simulink model "refroidissement_copy"  (R2019b)
settings: Solver=FixedStepAuto  StartTime=0.0  StopTime=inf  FixedStep=0.01  RelTol=1e-3
libraries: arduinolib x13, dspstat3 x6, simulink x2, LCDlib x1, Laboratoire x1
settings Model: SILPILModeSetting=veronly  ExtModeTrigDuration=2  Creator=Guy  LastModifiedBy=Etudiant
settings OptimizationCC: PassReuseOutputArgsAs=Individual arguments  ZeroExternalMemoryAtStartup=off  ZeroInternalMemoryAtStartup=off  MaxStackSize=64  OptimizeBlockOrder=speed  EfficientTunableParamExpr=on
settings DebuggingCC: ParameterTunabilityLossMsg=error
settings HardwareCC: ProdBitPerInt=16  ProdBitPerPointer=16  ProdBitPerSizeT=16  ProdBitPerPtrDiffT=16  ProdLargestAtomicFloat=None  ProdWordSize=8  ProdHWDeviceType=Atmel->AVR
settings SFSimCC: MATLABDynamicMemAlloc=off
settings RTWCC: SystemTargetFile=ert.tlc  HardwareBoard=Arduino Mega 2560  TLCOptions=-aInlineSetEventsForThisBaseRateFcn=TLC_FALSE -aSuppressMultiTaskScheduler=TLC_FALSE -aRateBasedStepFcn=1  TemplateMakefile=ert_default_tmf  CustomSource=enc_eml_src.c  Toolchain=Arduino AVR  BuildConfiguration=Faster Runs  IncludeHyperlinkInReport=on
settings CodeAppCC: ForceParamTrailComments=on  GenerateComments=off  IgnoreCustomStorageClasses=off  OperatorAnnotations=on  SimulinkDataObjDesc=on  SFDataObjDesc=on  InsertBlockDesc=on
settings ERTTargetCC: SupportContinuousTime=on  SupportVariableSizeSignals=on  ExtModeStaticAllocSize=2048

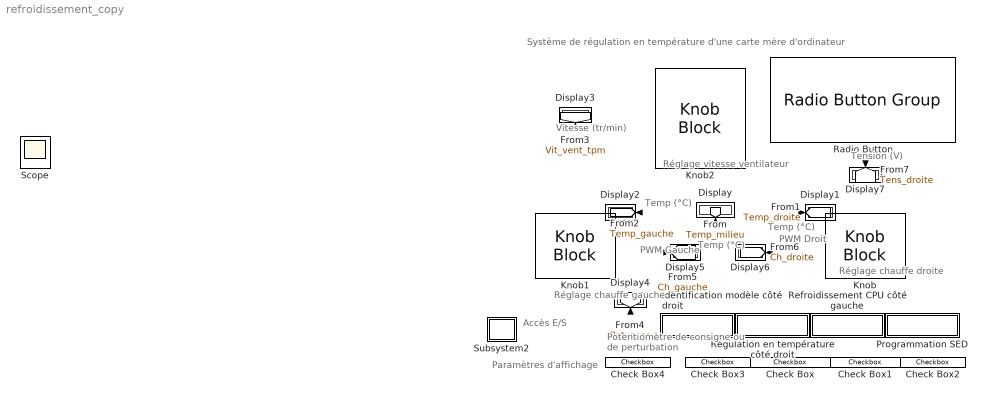
== system refroidissement_copy ==
  note: Paramètres d'affichage
  note: PWM
      | Gauche
  note: Système de régulation en température d'une carte mère d'ordinateur
  note: PWM
      | Droit
  note: Tension (V)
  note: Temp (°C)
  note: Temp (°C)
  note: Temp (°C)
  note: Vitesse (tr/min)
  note: Réglage vitesse ventilateur
  note: Réglage chauffe
      | droite
  note: Réglage chauffe
      | gauche
  note: Accès
      | E/S
  note: Potentiomètre
      | de consigne
      | ou de perturbation
  Check Box : Checkbox  LabelPosition=Hide  ShowInitialText=on  Label=Température gauche
  Check Box1 : Checkbox  LabelPosition=Hide  ShowInitialText=on  Label=Température milieu
  Check Box2 : Checkbox  LabelPosition=Hide  ShowInitialText=on  Label=Température droite
  Check Box3 : Checkbox  LabelPosition=Hide  ShowInitialText=on  Label=Tension résistance droite
  Check Box4 : Checkbox  LabelPosition=Hide  ShowInitialText=on  Label=Vitesse ventilateur (PWM)
  Display{,1..7} (8 alike) : Display
      Display3 settings: Decimation=20
  Identification modèle côté droit : Subsystem
  Knob : KnobBlock  LabelPosition=Hide  ScaleMax=255
  Knob1 : KnobBlock  LabelPosition=Hide  ScaleMax=255
  Knob2 : KnobBlock  LabelPosition=Hide  ScaleMax=255
  Programmation SED : Subsystem
  Radio Button : RadioButtonGroup  LabelPosition=Hide  SelectedLabel=Refroidissement CPU côté gauche  ButtonGroupName=Modes de marche
      settings: Values={{'Contrôle manuel', 'Régulation en température côté droit', 'Refroidissement CPU côté gauche', 'Programmation SED', 'Identification modèle côté droit', 'Arrêt'}, [0 1 2 3 4 5]}
  Refroidissement CPU côté gauche : Subsystem
  Régulation en température côté droit : Subsystem
  Subsystem2 : Subsystem
  Scope : Scope
  wires:
  [Temp_milieu] -> Display/1
  [Temp_droite] -> Display1/1
  [Temp_gauche] -> Display2/1
  [Vit_vent_tpm] -> Display3/1
  [Pot_cons] -> Display4/1
  [Ch_gauche] -> Display5/1
  [Ch_droite] -> Display6/1
  [Tens_droite] -> Display7/1

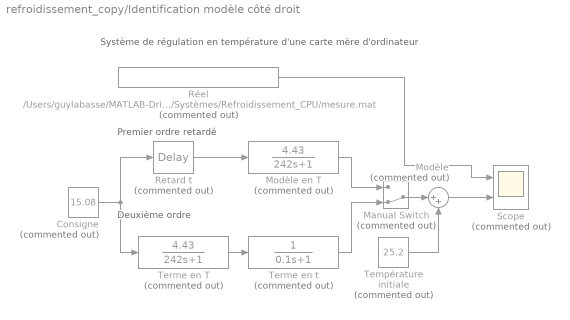
== system refroidissement_copy/Identification modèle côté droit ==
  note: Système de régulation en température d'une carte mère d'ordinateur
  note: Deuxième ordre
  note: Premier ordre retardé
  Consigne : Constant  Commented=on  Value=15.08
  Manual Switch : ManualSwitch  Commented=on  CurrentSetting=0
  Modèle : Sum  Commented=on  Inputs=|++
  Modèle en T : TransferFcn  Commented=on  Numerator=[4.43]  Denominator=[242 1]
  Retard t : TransportDelay  Commented=on  DelayTime=0.1
  Réel : FromFile  Commented=on  FileName=/Users/guylabasse/MATLAB-Drive/Systèmes/Refroidissement_CPU/mesure.mat  SampleTime=0.01
  Scope : Scope  Commented=on  NumInputPorts=2
  Température initiale : Constant  Commented=on  Value=25.2
  Terme en T : TransferFcn  Commented=on  Numerator=[4.43]  Denominator=[242 1]
  Terme en t : TransferFcn  Commented=on  Denominator=[0.1 1]
  wires:
  Consigne/1 -> Retard t/1, Terme en T/1
  Terme en T/1 -> Terme en t/1
  Température initiale/1 -> Modèle/2
  Terme en t/1 -> Manual Switch/2
  Modèle en T/1 -> Manual Switch/1
  Réel/1 -> Scope/1
  Manual Switch/1 -> Modèle/1
  Modèle/1 -> Scope/2
  Retard t/1 -> Modèle en T/1

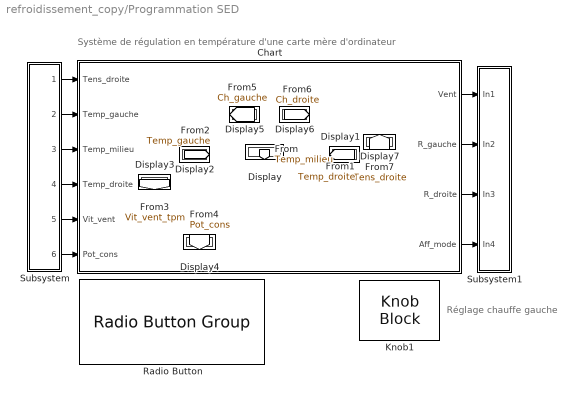
== system refroidissement_copy/Programmation SED ==
  note: Système de régulation en température d'une carte mère d'ordinateur
  note: Réglage chauffe
      | gauche
  Chart : Stateflow chart  BlockKeywords=__PRM__SERIALIZED__DATA__:Stateflow Chart,Stateflow Diagram  TreatAsAtomicUnit=on
  Display{,1..7} (8 alike) : Display
      Display3 settings: Decimation=20
  Knob1 : KnobBlock  LabelPosition=Hide  ScaleMax=250  TickInterval=50
  Radio Button : RadioButtonGroup  LabelPosition=Hide  SelectedLabel=Régulation en température côté gauche  ButtonGroupName=Modes de marche
      settings: Values={{'Contrôle manuel', 'Régulation en température côté droit', 'Régulation en température côté gauche', 'Programmation SED', 'Identification modèle côté droit', 'Arrêt'}, [0 1 2 3 4 5]}
  Subsystem : Subsystem
  Subsystem1 : Subsystem
  wires:
  [Temp_milieu] -> Display/1
  [Vit_vent_tpm] -> Display3/1
  [Tens_droite] -> Display7/1
  [Pot_cons] -> Display4/1
  [Temp_droite] -> Display1/1
  [Temp_gauche] -> Display2/1
  [Ch_gauche] -> Display5/1
  [Ch_droite] -> Display6/1
  Subsystem/1(Out1) -> Chart/1(Tens_droite)
  Subsystem/2(Out2) -> Chart/2(Temp_gauche)
  Subsystem/3(Out3) -> Chart/3(Temp_milieu)
  Subsystem/4(Out4) -> Chart/4(Temp_droite)
  Subsystem/5(Out5) -> Chart/5(Vit_vent)
  Subsystem/6(Out6) -> Chart/6(Pot_cons)
  Chart/1(Vent) -> Subsystem1/1(In1)
  Chart/2(R_gauche) -> Subsystem1/2(In2)
  Chart/3(R_droite) -> Subsystem1/3(In3)
  Chart/4(Aff_mode) -> Subsystem1/4(In4)

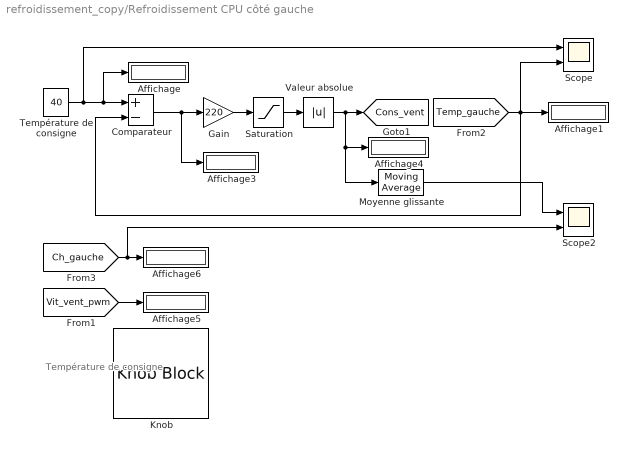
== system refroidissement_copy/Refroidissement CPU côté gauche ==
  note: Température
      | de consigne
  Affichage{,1,3..6} (6 alike) : Display
  Comparateur : Sum  Inputs=+-  OutDataTypeStr=double
  Gain : Gain  Gain=220
  Knob : KnobBlock  LabelPosition=Hide  TickInterval=10
  Moyenne glissante : dspstat3/Moving Average  Method=Sliding window  ForgettingFactorPort=off  SpecifyWindowLength=on  WindowLength=20  ForgettingFactor=0.9  SimulateUsing=Code generation
  Saturation : Saturate  UpperLimit=-81  LowerLimit=-10000
  Scope : Scope  NumInputPorts=2
  Scope2 : Scope  NumInputPorts=2
  Température de consigne : Constant  Value=40  SampleTime=-1
  Valeur absolue : Abs
  tag scope: Cons_vent=global
  wires:
  Température de consigne/1 -> Scope/1, Comparateur/1, Affichage/1
  Comparateur/1 -> Gain/1, Affichage3/1
  [Temp_gauche] -> Scope/2, Affichage1/1, Comparateur/2
  Gain/1 -> Saturation/1
  Valeur absolue/1 -> Affichage4/1, Moyenne glissante/1, [Cons_vent]
  [Vit_vent_pwm] -> Affichage5/1
  [Ch_gauche] -> Scope2/2, Affichage6/1
  Saturation/1 -> Valeur absolue/1
  Moyenne glissante/1 -> Scope2/1

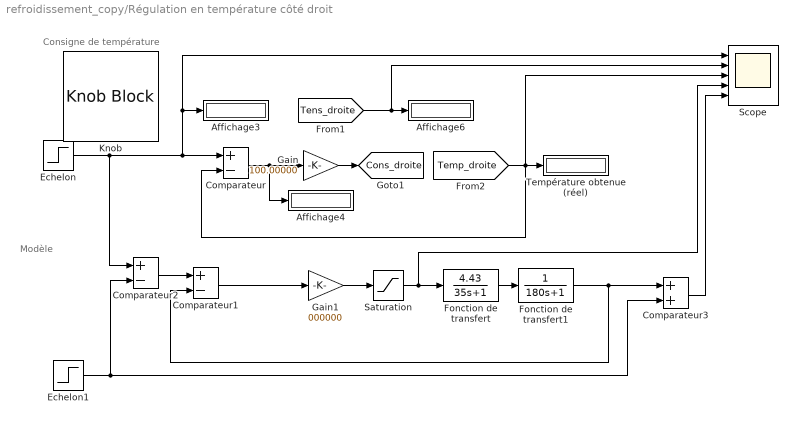
== system refroidissement_copy/Régulation en température côté droit ==
  note: Modèle
  note: Consigne de température
  Affichage3 : Display
  Affichage4 : Display
  Affichage6 : Display
  Comparateur : Sum  Inputs=+-  OutDataTypeStr=double
  Comparateur1 : Sum  Inputs=+-  OutDataTypeStr=double
  Comparateur2 : Sum  Inputs=+-  OutDataTypeStr=double
  Comparateur3 : Sum  OutDataTypeStr=double
  Echelon : Step  Time=0  After=0
  Echelon1 : Step  Time=10  After=0
  Fonction de transfert : TransferFcn  Numerator=[4.43]  Denominator=[35 1]
  Fonction de transfert1 : TransferFcn  Denominator=[180 1]
  Gain : Gain  Gain=100.00000
  Gain1 : Gain  Gain=000000
  Knob : KnobBlock  LabelPosition=Hide  TickInterval=20
  Saturation : Saturate  UpperLimit=15.08  LowerLimit=0
  Scope : Scope  NumInputPorts=5
  Température obtenue (réel) : Display
  tag scope: Cons_droite=global
  wires:
  [Tens_droite] -> Scope/2, Affichage6/1
  Echelon/1 -> Comparateur/1, Affichage3/1, Scope/1, Comparateur2/1
  [Temp_droite] -> Scope/3, Température obtenue (réel)/1, Comparateur/2
  Comparateur/1 -> Affichage4/1, Gain/1
  Gain/1 -> [Cons_droite]
  Comparateur1/1 -> Gain1/1
  Comparateur2/1 -> Comparateur1/1
  Echelon1/1 -> Comparateur3/2, Comparateur2/2
  Saturation/1 -> Scope/4, Fonction de transfert/1
  Fonction de transfert/1 -> Fonction de transfert1/1
  Fonction de transfert1/1 -> Comparateur1/2, Comparateur3/1
  Comparateur3/1 -> Scope/5
  Gain1/1 -> Saturation/1

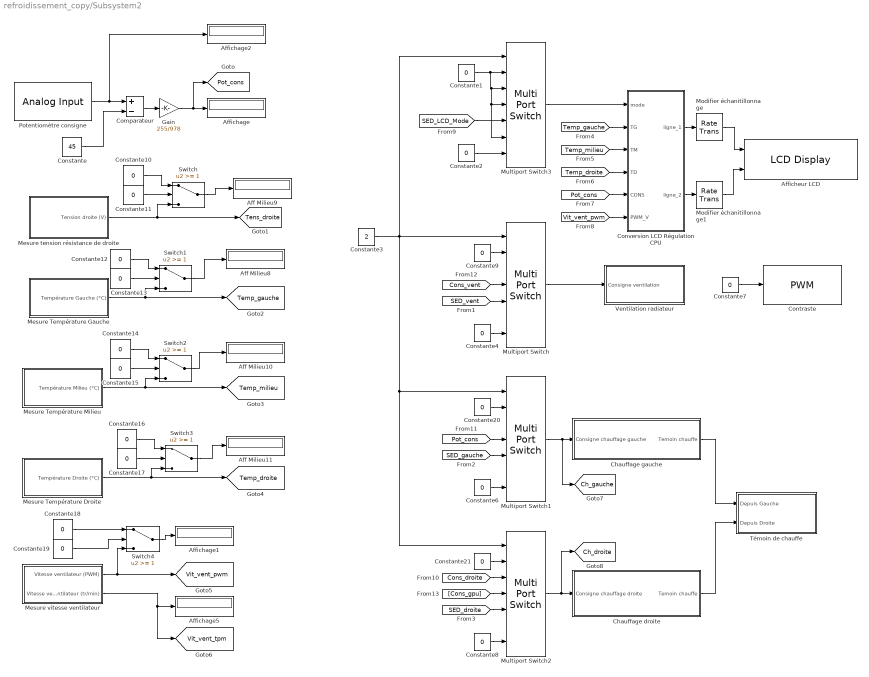
== system refroidissement_copy/Subsystem2 ==
  Aff Milieu{8..11} (4 alike) : Display
  Affichage{,1..2,5} (4 alike) : Display
  Afficheur LCD : LCDlib/LCD Display  pins=[30, 31, 32, 34, 36, 38]
      settings: SourceProductName=Arduino Extra Library
  Chauffage droite : Subsystem
  Chauffage gauche : Subsystem
  Comparateur : Sum  Inputs=+-  OutDataTypeStr=double
  Constante : Constant  Value=45  SampleTime=-1
  Constante{1..2,4,6,8..21} (18 alike) : Constant  Value=0  SampleTime=-1
  Constante3 : Constant  Value=2  SampleTime=-1
  Constante7 : Constant  Value=0  OutDataTypeStr=uint16  SampleTime=-1
  Contraste : arduinolib/PWM  pinNumber=44  EnableInputFrequency=off  InitialFrequency=2000  InitialDutyCycle=0  NotificationType=None  blockPlatform=arduino
  Conversion LCD Régulation CPU : MATLAB Function  TreatAsAtomicUnit=on
  Gain : Gain  Gain=255/978
  Mesure Température Droite : Subsystem
  Mesure Température Gauche : Subsystem
  Mesure Température Milieu : Subsystem
  Mesure tension résistance de droite : Subsystem
  Mesure vitesse ventilateur : Subsystem
  Modifier échanitillonnage : RateTransition  Integrity=off  OutPortSampleTime=1
  Modifier échanitillonnage1 : RateTransition  Integrity=off  OutPortSampleTime=1
  Multiport Switch{,1..3} (4 alike) : MultiPortSwitch  DataPortOrder=Zero-based contiguous  Inputs=6  DiagnosticForDefault=None  zeroidx=on  OutDataTypeStr=double
  Potentiomètre consigne : arduinolib/Analog Input  pinNumber=3  ReadResultsOnly=off  ConversionTriggerSource=Software  ExternalTriggerType=uint32(0)  OutputDataType=uint16  EnableConversionCompleteNotify=off  EnableOuputStatus=off  SampleTime=-1  blockPlatform=arduino
  Switch{,1..4} (5 alike) : Switch  Threshold=1
  Témoin de chauffe : Subsystem
  Ventilation radiateur : Subsystem
  tag scope: Ch_droite=global, Ch_gauche=global, Pot_cons=global, Temp_droite=global, Temp_gauche=global, Temp_milieu=global, Tens_droite=global, Vit_vent_pwm=global, Vit_vent_tpm=global
  wires:
  Modifier échanitillonnage1/1 -> Afficheur LCD/2
  Modifier échanitillonnage/1 -> Afficheur LCD/1
  Conversion LCD Régulation CPU/1(ligne_1) -> Modifier échanitillonnage/1
  Conversion LCD Régulation CPU/2(ligne_2) -> Modifier échanitillonnage1/1
  Mesure vitesse ventilateur/2(Vitesse ventilateur (tr/min)) -> [Vit_vent_tpm], Affichage5/1
  Mesure vitesse ventilateur/1(Vitesse ventilateur (PWM)) -> Switch4/3, [Vit_vent_pwm]
  Constante7/1 -> Contraste/1
  Multiport Switch/1 -> Ventilation radiateur/1(Consigne ventilation)
  Multiport Switch2/1 -> Chauffage droite/1(Consigne chauffage droite), [Ch_droite]
  Chauffage gauche/1(Temoin chauffe) -> Témoin de chauffe/1(Depuis Gauche)
  Multiport Switch1/1 -> [Ch_gauche], Chauffage gauche/1(Consigne chauffage gauche)
  Chauffage droite/1(Temoin chauffe) -> Témoin de chauffe/2(Depuis Droite)
  Gain/1 -> [Pot_cons], Affichage/1
  Switch/1 -> Aff Milieu9/1
  Mesure tension résistance de droite/1(Tension droite (V)) -> [Tens_droite], Switch/3
  Constante10/1 -> Switch/1
  Constante11/1 -> Switch/2
  Constante12/1 -> Switch1/1
  Constante13/1 -> Switch1/2
  Mesure Température Gauche/1(Température Gauche (°C)) -> [Temp_gauche], Switch1/3
  Switch1/1 -> Aff Milieu8/1
  Constante14/1 -> Switch2/1
  Constante15/1 -> Switch2/2
  Mesure Température Milieu/1(Température Milieu (°C)) -> [Temp_milieu], Switch2/3
  Switch2/1 -> Aff Milieu10/1
  Constante16/1 -> Switch3/1
  Constante17/1 -> Switch3/2
  Mesure Température Droite/1(Température Droite (°C)) -> [Temp_droite], Switch3/3
  Switch3/1 -> Aff Milieu11/1
  Constante18/1 -> Switch4/1
  Constante19/1 -> Switch4/2
  Switch4/1 -> Affichage1/1
  Constante4/1 -> Multiport Switch/7
  Constante6/1 -> Multiport Switch1/7
  Constante8/1 -> Multiport Switch2/7
  Constante3/1 -> Multiport Switch3/1, Multiport Switch/1, Multiport Switch1/1, Multiport Switch2/1
  Constante9/1 -> Multiport Switch/2
  Constante20/1 -> Multiport Switch1/2
  Constante21/1 -> Multiport Switch2/2
  [SED_vent] -> Multiport Switch/5
  [SED_gauche] -> Multiport Switch1/5
  [SED_droite] -> Multiport Switch2/5
  Multiport Switch3/1 -> Conversion LCD Régulation CPU/1(mode)
  Constante1/1 -> Multiport Switch3/6, Multiport Switch3/4, Multiport Switch3/3, Multiport Switch3/2
  Constante2/1 -> Multiport Switch3/7
  [Temp_gauche] -> Conversion LCD Régulation CPU/2(TG)
  [Temp_milieu] -> Conversion LCD Régulation CPU/3(TM)
  [Temp_droite] -> Conversion LCD Régulation CPU/4(TD)
  [Pot_cons] -> Conversion LCD Régulation CPU/5(CONS)
  [Vit_vent_pwm] -> Conversion LCD Régulation CPU/6(PWM_V)
  [SED_LCD_Mode] -> Multiport Switch3/5
  [Cons_droite] -> Multiport Switch2/3
  [Cons_vent] -> Multiport Switch/4
  [Pot_cons] -> Multiport Switch1/4
  [Cons_gpu] -> Multiport Switch2/4
  Comparateur/1 -> Gain/1
  Potentiomètre consigne/1 -> Affichage2/1, Comparateur/1
  Constante/1 -> Comparateur/2

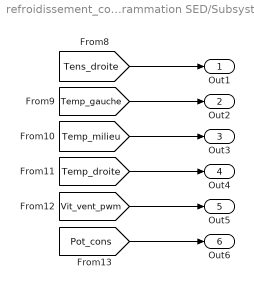
== system refroidissement_copy/Programmation SED/Subsystem ==
  Out1 : Outport
  Out2 : Outport  Port=2
  Out3 : Outport  Port=3
  Out4 : Outport  Port=4
  Out5 : Outport  Port=5
  Out6 : Outport  Port=6
  wires:
  [Temp_milieu] -> Out3/1
  [Vit_vent_pwm] -> Out5/1
  [Temp_droite] -> Out4/1
  [Tens_droite] -> Out1/1
  [Temp_gauche] -> Out2/1
  [Pot_cons] -> Out6/1

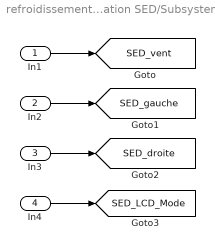
== system refroidissement_copy/Programmation SED/Subsystem1 ==
  In1 : Inport
  In2 : Inport  Port=2
  In3 : Inport  Port=3
  In4 : Inport  Port=4
  tag scope: SED_LCD_Mode=global, SED_droite=global, SED_gauche=global, SED_vent=global
  wires:
  In2/1 -> [SED_gauche]
  In4/1 -> [SED_LCD_Mode]
  In1/1 -> [SED_vent]
  In3/1 -> [SED_droite]

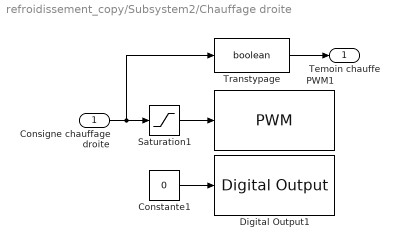
== system refroidissement_copy/Subsystem2/Chauffage droite ==
  Consigne chauffage droite : Inport
  Constante1 : Constant  Value=0  SampleTime=-1
  Digital Output1 : arduinolib/Digital Output  pinNumber=10  blockPlatform=arduino
  PWM1 : arduinolib/PWM  pinNumber=7  EnableInputFrequency=off  InitialFrequency=2000  InitialDutyCycle=0  NotificationType=None  blockPlatform=arduino
  Saturation1 : Saturate  UpperLimit=255  LowerLimit=0
  Transtypage : DataTypeConversion  OutDataTypeStr=boolean
  Temoin chauffe : Outport  VectorParamsAs1DForOutWhenUnconnected=off
  wires:
  Saturation1/1 -> PWM1/1
  Constante1/1 -> Digital Output1/1
  Consigne chauffage droite/1 -> Transtypage/1, Saturation1/1
  Transtypage/1 -> Temoin chauffe/1

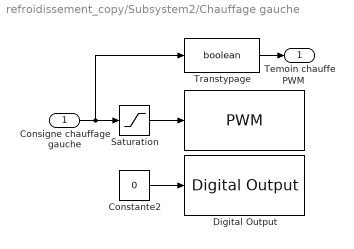
== system refroidissement_copy/Subsystem2/Chauffage gauche ==
  Consigne chauffage gauche : Inport
  Constante2 : Constant  Value=0  SampleTime=-1
  Digital Output : arduinolib/Digital Output  pinNumber=9  blockPlatform=arduino
  PWM : arduinolib/PWM  pinNumber=6  EnableInputFrequency=off  InitialFrequency=2000  InitialDutyCycle=0  NotificationType=None  blockPlatform=arduino
  Saturation : Saturate  UpperLimit=255  LowerLimit=0
  Transtypage : DataTypeConversion  OutDataTypeStr=boolean
  Temoin chauffe : Outport  VectorParamsAs1DForOutWhenUnconnected=off
  wires:
  Constante2/1 -> Digital Output/1
  Saturation/1 -> PWM/1
  Consigne chauffage gauche/1 -> Transtypage/1, Saturation/1
  Transtypage/1 -> Temoin chauffe/1

== system refroidissement_copy/Subsystem2/Mesure Température Droite ==
  Gain2 : Gain  Gain=27.2/238.4
  Mesure Température droite : arduinolib/Analog Input  pinNumber=2  ReadResultsOnly=off  ConversionTriggerSource=Software  ExternalTriggerType=uint32(0)  OutputDataType=uint16  EnableConversionCompleteNotify=off  EnableOuputStatus=off  SampleTime=-1  blockPlatform=arduino
  Moyenne Droite : dspstat3/Moving Average  Method=Sliding window  ForgettingFactorPort=off  SpecifyWindowLength=on  WindowLength=5  ForgettingFactor=0.9  SimulateUsing=Code generation
  Transtypage3 : DataTypeConversion  OutDataTypeStr=double
  Température Droite (°C) : Outport
  wires:
  Gain2/1 -> Moyenne Droite/1
  Moyenne Droite/1 -> Température Droite (°C)/1
  Mesure Température droite/1 -> Transtypage3/1
  Transtypage3/1 -> Gain2/1

== system refroidissement_copy/Subsystem2/Mesure Température Gauche ==
  Gain : Gain  Gain=27.2/238.2
  Mesure Température gauche : arduinolib/Analog Input  pinNumber=0  ReadResultsOnly=off  ConversionTriggerSource=Software  ExternalTriggerType=uint32(0)  OutputDataType=uint16  EnableConversionCompleteNotify=off  EnableOuputStatus=off  SampleTime=-1  blockPlatform=arduino
  Moyenne Gauche : dspstat3/Moving Average  Method=Sliding window  ForgettingFactorPort=off  SpecifyWindowLength=on  WindowLength=5  ForgettingFactor=0.9  SimulateUsing=Code generation
  Transtypage1 : DataTypeConversion  OutDataTypeStr=double
  Température Gauche (°C) : Outport
  wires:
  Gain/1 -> Moyenne Gauche/1
  Mesure Température gauche/1 -> Transtypage1/1
  Transtypage1/1 -> Gain/1
  Moyenne Gauche/1 -> Température Gauche (°C)/1

== system refroidissement_copy/Subsystem2/Mesure Température Milieu ==
  Gain1 : Gain  Gain=27.2/234.8
  Mesure Température milieu : arduinolib/Analog Input  pinNumber=1  ReadResultsOnly=off  ConversionTriggerSource=Software  ExternalTriggerType=uint32(0)  OutputDataType=uint16  EnableConversionCompleteNotify=off  EnableOuputStatus=off  SampleTime=-1  blockPlatform=arduino
  Moyenne Milieu : dspstat3/Moving Average  Method=Sliding window  ForgettingFactorPort=off  SpecifyWindowLength=on  WindowLength=5  ForgettingFactor=0.9  SimulateUsing=Code generation
  Transtypage2 : DataTypeConversion  OutDataTypeStr=double
  Température Milieu (°C) : Outport
  wires:
  Gain1/1 -> Moyenne Milieu/1
  Mesure Température milieu/1 -> Transtypage2/1
  Transtypage2/1 -> Gain1/1
  Moyenne Milieu/1 -> Température Milieu (°C)/1

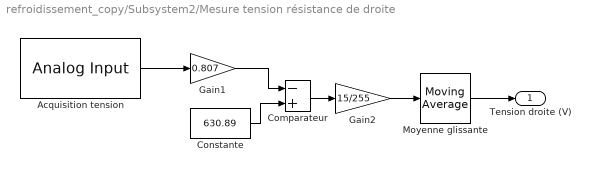
== system refroidissement_copy/Subsystem2/Mesure tension résistance de droite ==
  Acquisition tension : arduinolib/Analog Input  pinNumber=4  ReadResultsOnly=off  ConversionTriggerSource=Software  ExternalTriggerType=uint32(0)  OutputDataType=uint16  EnableConversionCompleteNotify=off  EnableOuputStatus=off  SampleTime=-1  blockPlatform=arduino
  Comparateur : Sum  Inputs=-+  OutDataTypeStr=double
  Constante : Constant  Value=630.89  SampleTime=-1
  Gain1 : Gain  Gain=0.807
  Gain2 : Gain  Gain=15/255
  Moyenne glissante : dspstat3/Moving Average  Method=Sliding window  ForgettingFactorPort=off  SpecifyWindowLength=on  WindowLength=4  ForgettingFactor=0.9  SimulateUsing=Code generation
  Tension droite (V) : Outport
  wires:
  Acquisition tension/1 -> Gain1/1
  Gain2/1 -> Moyenne glissante/1
  Constante/1 -> Comparateur/2
  Comparateur/1 -> Gain2/1
  Moyenne glissante/1 -> Tension droite (V)/1
  Gain1/1 -> Comparateur/1

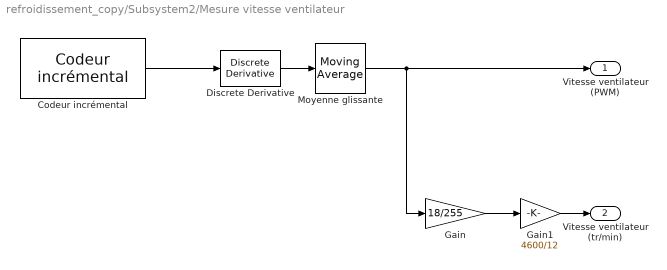
== system refroidissement_copy/Subsystem2/Mesure vitesse ventilateur ==
  Codeur incrémental : Laboratoire/Arduino/Codeur incrémental  enc=0  pinA=2  pinB=2  T=-1
      settings: SourceProductName=Laboratoire Dautet
  Discrete Derivative : simulink/Discrete/Discrete Derivative  gainval=1.0  ICPrevScaledInput=0.0  OutMin=[]  OutMax=[]  OutDataType=fixdt(1, 16)  OutScaling=2^-10  DoSatur=off
  Gain : Gain  Gain=18/255
  Gain1 : Gain  Gain=4600/12
  Moyenne glissante : dspstat3/Moving Average  Method=Sliding window  ForgettingFactorPort=off  SpecifyWindowLength=on  WindowLength=5  ForgettingFactor=0.9  SimulateUsing=Code generation
  Vitesse ventilateur (PWM) : Outport
  Vitesse ventilateur (tr/min) : Outport  Port=2
  wires:
  Discrete Derivative/1 -> Moyenne glissante/1
  Moyenne glissante/1 -> Vitesse ventilateur (PWM)/1, Gain/1
  Codeur incrémental/1 -> Discrete Derivative/1
  Gain/1 -> Gain1/1
  Gain1/1 -> Vitesse ventilateur (tr/min)/1

== system refroidissement_copy/Subsystem2/Témoin de chauffe ==
  Depuis Gauche : Inport
  Depuis Droite : Inport  Port=2
  Générateur signal : DiscretePulseGenerator  PulseType=Time based  Amplitude=255  PulseWidth=50
  Led : arduinolib/PWM  pinNumber=11  EnableInputFrequency=off  InitialFrequency=2000  InitialDutyCycle=0  NotificationType=None  blockPlatform=arduino
  Opérateur logique : Logic  Operator=OR  AllPortsSameDT=off  OutDataTypeStr=boolean
  Produit : Product
  wires:
  Depuis Gauche/1 -> Opérateur logique/1
  Depuis Droite/1 -> Opérateur logique/2
  Opérateur logique/1 -> Produit/1
  Générateur signal/1 -> Produit/2
  Produit/1 -> Led/1

== system refroidissement_copy/Subsystem2/Ventilation radiateur ==
  Consigne ventilation : Inport
  Commande MOS : arduinolib/PWM  pinNumber=8  EnableInputFrequency=off  InitialFrequency=2000  InitialDutyCycle=0  NotificationType=None  blockPlatform=arduino
  Comparer à constante : simulink/Logic and Bit Operations/Compare To Constant  relop=>=  const=80  OutDataTypeStr=boolean
  Gain : Gain  Gain=255
  PWM Ventirad : arduinolib/PWM  pinNumber=12  EnableInputFrequency=off  InitialFrequency=2000  InitialDutyCycle=0  NotificationType=None  blockPlatform=arduino
  Transtypage : DataTypeConversion  OutDataTypeStr=boolean
  wires:
  Consigne ventilation/1 -> Comparer à constante/1, PWM Ventirad/1
  Transtypage/1 -> Gain/1
  Gain/1 -> Commande MOS/1
  Comparer à constante/1 -> Transtypage/1

== matlab function refroidissement_copy/Subsystem2/Conversion LCD Régulation CPU ==
  data: mode input double; TG input size=1; ligne_1 output uint8 size=1 16; TM input; TD input; CONS input; PWM_V input; ligne_2 output
function [ligne_1,ligne_2] = fcn(mode, TG, TM, TD, CONS, PWM_V)

% Guy Labasse - Lycée Dautet 2019
% Modifié pour TP Régulation CPU

% mode == 0 --> Test Afficheur
% mode == 1 --> température
% mode == 2 --> 
% mode == 3 --> 
% mode == 4 --> 
% mode == 5 --> 
% mode == 6 --> 
% mode == 7 --> Bienvenue ...
% Toute autre valeur de mode --> Erreur !

% val: valeur numérique réel double précision

% La fonction décode de 000 à 999
% Toute valeur au delà sera saturée à 999

ligne_1= uint8(zeros([1 16]));
ligne_2= uint8(zeros([1 16]));
valeur              = single(TG);
mode                = uint8(mode);




%% Gestion du mode d'ligne_1
if mode == 0
    ligne_1(1:16)      = uint8([82 101 102 114 111 105 100 105 115 115 101 109 101 110 116 32]);
    ligne_2(1:16)      = uint8([80 114 111 99 101 115 115 101 117 114 32 51 53 32 87 32]);
elseif mode == 1
    ligne_1(1:7)      = uint8([84   101   109   112    58    32   32]);
    ligne_1([14 15 16])  = uint8([32 67 32]);
elseif mode == 2
    ligne_1(1:7)      = uint8([72   117   109   105    58    32   32]);
    ligne_1([14 15 16])  = uint8([32 37 32]);
elseif mode == 3
    ligne_1(1:7)      = uint8([77   97   115   115    101    58   32]);
    ligne_1([14 15 16])  = uint8([32 103 32]);
elseif mode == 4
    ligne_1(1:7)      = uint8([86   111   108   117    109    101   58]);
    ligne_1([14 15 16])  = uint8([32 109 108]);
elseif mode == 5
    ligne_1(1:16)      = uint8([84 80 32 66 97 108 97 110 99 101 32 72 97 108 111 32]);
elseif mode == 6
    ligne_1(1:16)      = uint8([45 45 45 45 32 32 32 32 32 32 32 32 32 32 32 32]);
elseif mode == 7
    ligne_1(1:16)      = uint8([66 105 101 110 118 101 110 117 101 32 46 46 46 32 32 32]);
else
    ligne_1(1:16)      = uint8([69 114 114 101 117 114 32 33 32 32 32 32 32 32 32 32]);
end

end

function titi = affichevaleur(valeur,pos,ligne_1)
%% ligne_1 sur trois caractères

% Premier caratère (centaines)
v           = fix(valeur);
a           = abs(v);

if a>=0 && a<100
    ligne_1(9)    = uint8(48);
    b       = a;
    
elseif a>=100 && a<200
    ligne_1(9)    = uint8(49);
    b       = a-100;
    
elseif a>=200 && a<300
    ligne_1(9)    = uint8(50);
    b       = a-200;
    
elseif a>=300 && a<400
    ligne_1(9)    = uint8(51);
    b       = a-300;
    
elseif a>=400 && a<500
    ligne_1(9)    = uint8(52);
    b       = a-400;
    
elseif a>=500 && a<600
    ligne_1(9)    = uint8(53);
    b       = a-500;
    
elseif a>=600 && a<700
    ligne_1(9)    = uint8(54);
    b       = a-600;
    
elseif a>=700 && a<800
    ligne_1(9)    = uint8(55);
    b       = a-700;
    
elseif a>=800 && a<900
    ligne_1(9)    = uint8(56);
    b       = a-800;
    
elseif a>=900 && a<1000
    ligne_1(9)    = uint8(57);
    b       = a-900;
    
else
    ligne_1(9)    = uint8(57);
    b       = single(99);
end

% Deuxième caratère (dizaines)

if b>=0 && b<10
    ligne_1(10)    = uint8(48);
    c       = b;
    
elseif b>=10 && b<20
    ligne_1(10)    = uint8(49);
    c       = b-10;
    
elseif b>=20 && b<30
    ligne_1(10)    = uint8(50);
    c       = b-20;
    
elseif b>=30 && b<40
    ligne_1(10)    = uint8(51);
    c       = b-30;
    
elseif b>=40 && b<50
    ligne_1(10)    = uint8(52);
    c       = b-40;
    
elseif b>=50 && b<60
    ligne_1(10)    = uint8(53);
    c       = b-50;
    
elseif b>=60 && b<70
    ligne_1(10)    = uint8(54);
    c       = b-60;
    
elseif b>=70 && b<80
    ligne_1(10)    = uint8(55);
    c       = b-70;
    
elseif b>=80 && b<90
    ligne_1(10)    = uint8(56);
    c       = b-80;
    
elseif b>=90 && b<100
    ligne_1(10)    = uint8(57);
    c       = b-90;
    
else
    ligne_1(10)    = uint8(57);
    c       = single(9);
end

% Troisième caratère (unités)
ligne_1(11)        = determineNombre(c);
end
%% ligne_1 Ascii des caractères

function d = determineNombre(n)

    switch n
        case 0
            d = uint8(48);
        case 1
            d = uint8(49);
        case 2
            d = uint8(50);
        case 3
            d = uint8(51);
        case 4
            d = uint8(52);
        case 5
            d = uint8(53);
        case 6
            d = uint8(54);
        case 7
            d = uint8(55);
        case 8
            d = uint8(56);
        case 9
            d = uint8(57);    
        otherwise
            d = uint8(57);
    end

end

== stateflow chart refroidissement_copy/Programmation SED/Chart ==
  data: Tens_droite input; Temp_gauche input; Temp_milieu input; Temp_droite input; Vit_vent input; Pot_cons input; Vent output double; R_gauche output double; R_droite output double; Aff_mode output double
